simulink model "cartesian_regulation_crl"  (R2025b)
settings: Solver=VariableStepAuto  StartTime=0.0  StopTime=10  RelTol=1e-3
libraries: robotmobilelib x1
settings Model: Creator=alessandrochinello  LastModifiedBy=mattc

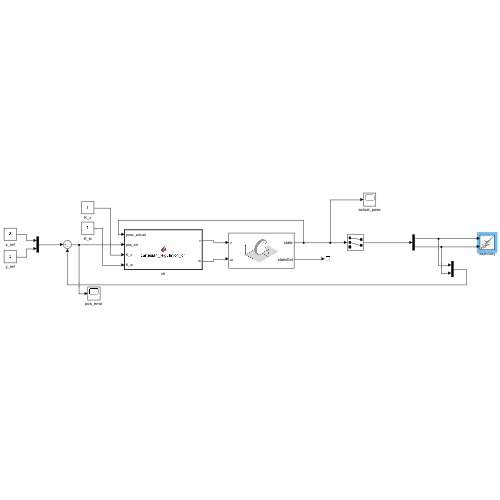
[thumbnail: Simulink's stored preview of the top-level diagram]
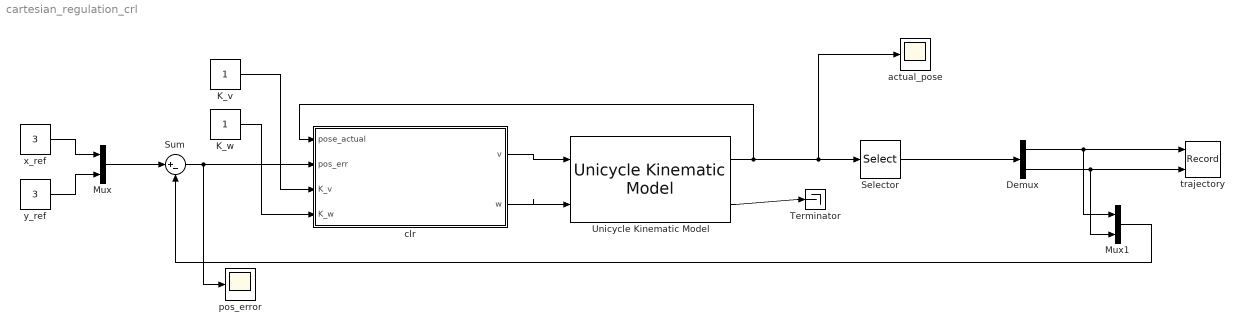
== system cartesian_regulation_crl ==
  Demux : Demux  Outputs=2
  K_v : Constant
  K_w : Constant
  Mux : Mux  Inputs=2
  Mux1 : Mux  Inputs=2
  Selector : Selector  InputPortWidth=3  IndexOptions=Index vector (dialog)  Indices=[1 2]  OutputSizes=1
  Sum : Sum  Inputs=|+-
  Terminator : Terminator
  Unicycle Kinematic Model : robotmobilelib/Unicycle Kinematic Model  VehicleInputs=Vehicle Speed & Heading Angular Velocity  WheelRadius=0.1  WheelSpeedRange=[-Inf Inf]  InitialState=[0; 0; 0]  SimulateUsing=Interpreted execution
  actual_pose : Scope
      settings: ActiveDisplayYMinimum=-226.27478329942264  ActiveDisplayYMaximum=95.764724549776915
  clr : MATLAB Function  TreatAsAtomicUnit=on
  pos_error : Scope
      settings: ActiveDisplayYMinimum=-226.27478329942264  ActiveDisplayYMaximum=95.764724549776915
  trajectory : Record  NumPorts=2.0  FileSettingsInternal="{\"entries\":[{\"content\":{\"excelSettings\":{\"content\":{},\"type\":\"Streamout.ExcelSettings\"},\"parquetSettings\":{\"content\":{},\"type\":\"Streamout.ParquetSettings\"}},\"type\":\"Streamout.FileSettingStorage\",\"uuid\":\"\"}],\"packageUris\":[\"http:\\/\\/schema.mathworks.com\\/mf0\\/streamout_blocks\\/R2020a\"],\"version\":\"1.0\"}"  FrameSettings=[0, 0]  Layout=[1 1]  SignalsInternal="{\"entries\":[{\"content\":{\"signals\":[{\"content\":{\"blockPath\":[],\"dimensions\":[1],\"domain\":\"\",\"lineColor\":\"#a2142f\",\"plots\":[ 1 ],\"port\":1,\"sid\":[\"\"],\"signalID\":1,\"signalName\":\"Demux:1\"},\"type\":\"RecordBlkView.Signal\",\"uuid\":\"\"},{\"content\":{\"blockPath\":[],\"dimensions\":[1],\"domain\":\"\",\"lineColor\":\"#139fff\",\"plots\":[ 1 ],\"port\":2,\"sid\":[\"\"],\"signalID\":2,\"signalName\":\"Demux:2\"},\"type\":\"RecordBlkView.Signal\",\"uuid\":\"\"}]},\"type\":\"RecordBlkView.InputSignals\",\"uuid\":\"\"}],\"packageUris\":[\"http:\\/\\/schema.mathworks.com\\/mf0\\/streamout_blocks\\/R2020a\"],\"version\":\"1.0\"}"  VisualizationBindings="{\"xyplotplugin\":{\"info\":[{\"series\":[{\"bindingParametersList\":[{\"parameter\":\"X-Axis\",\"signalID\":1,\"signalName\":\"Demux:1\"},{\"parameter\":\"Y-Axis\",\"signalID\":2,\"signalName\":\"Demux:2\"}],\"seriesID\":0}],\"subplotID\":1}]}}"  CompatibilityTag=XY
  x_ref : Constant  Value=3
  y_ref : Constant  Value=3
  wires:
  clr/2(w) -> Unicycle Kinematic Model/2
  clr/1(v) -> Unicycle Kinematic Model/1
  x_ref/1 -> Mux/1
  y_ref/1 -> Mux/2
  Mux/1 -> Sum/1
  Unicycle Kinematic Model/1 -> clr/1(pose_actual), actual_pose/1, Selector/1
  K_v/1 -> clr/3(K_v)
  K_w/1 -> clr/4(K_w)
  Unicycle Kinematic Model/2 -> Terminator/1
  Sum/1 -> pos_error/1, clr/2(pos_err)
  Demux/1 -> Mux1/1, trajectory/1
  Demux/2 -> trajectory/2, Mux1/2
  Mux1/1 -> Sum/2
  Selector/1 -> Demux/1

== matlab function cartesian_regulation_crl/clr ==
  data: pose_actual input; pos_err input; v output; w output; K_v input; K_w input
function [v, w] = cartesian_regulation_crl(pose_actual, pos_err, K_v, K_w)

x = pose_actual(1);
y = pose_actual(2);
theta = pose_actual(3);

n = [cos(theta); sin(theta)];
gamma = wrapToPi(atan2(pos_err(2), pos_err(1)) - theta);


v = K_v * dot(pos_err, n);
w = K_w * gamma;

end
